simulink model "motorV1"  (R2022b)
settings: Solver=VariableStepAuto  StartTime=0.0  StopTime=10.0  RelTol=1e-3
undefined symbols (not defined in the file or in its folder): flux_a, flux_b, flux_c, Fx_idq, Fy_idq
settings Model: Creator=ramuj  LastModifiedBy=ramuj

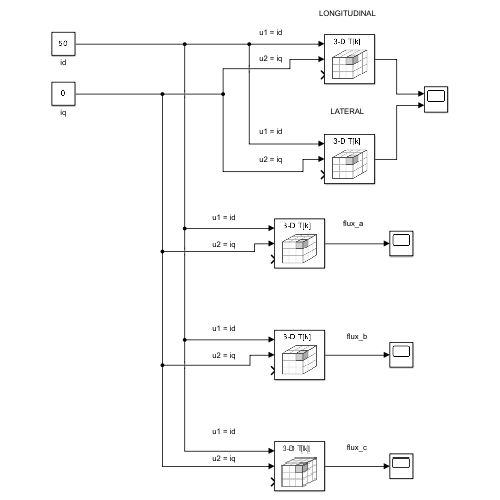
[thumbnail: Simulink's stored preview of the top-level diagram]
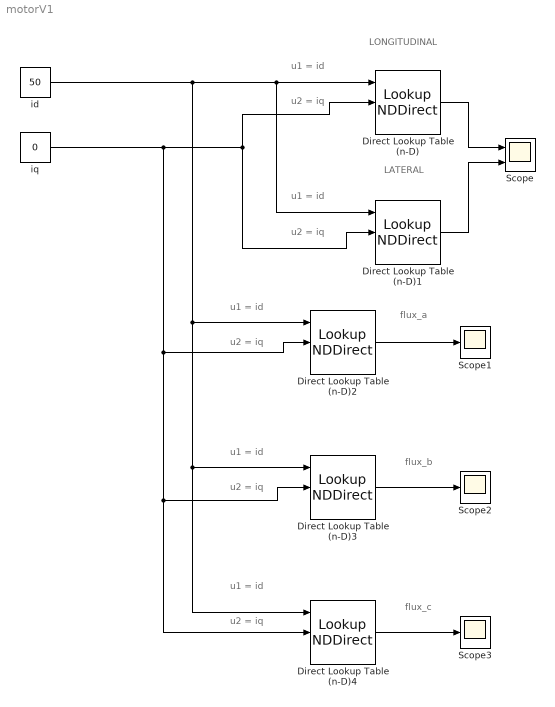
== system motorV1 ==
  note: flux_a
  note: u2 = iq
  note: u1 = id
  note: LONGITUDINAL
  note: LATERAL
  note: u1 = id
  note: u2 = iq
  note: u1 = id
  note: u2 = iq
  note: u2 = iq
  note: flux_b
  note: u1 = id
  note: flux_c
  note: u2 = iq
  note: u1 = id
  Direct Lookup Table (n-D) : LookupNDDirect  NumberOfTableDimensions=3  Table=Fx_idq
  Direct Lookup Table (n-D)1 : LookupNDDirect  NumberOfTableDimensions=3  Table=Fy_idq
  Direct Lookup Table (n-D)2 : LookupNDDirect  NumberOfTableDimensions=3  Table=flux_a
  Direct Lookup Table (n-D)3 : LookupNDDirect  NumberOfTableDimensions=3  Table=flux_b
  Direct Lookup Table (n-D)4 : LookupNDDirect  NumberOfTableDimensions=3  Table=flux_c
  Scope : Scope  NumInputPorts=2
  Scope1 : Scope
  Scope2 : Scope
  Scope3 : Scope
  id : Constant  Value=50
  iq : Constant  Value=0
  wires:
  Direct Lookup Table (n-D)/1 -> Scope/1
  Direct Lookup Table (n-D)1/1 -> Scope/2
  Direct Lookup Table (n-D)2/1 -> Scope1/1
  Direct Lookup Table (n-D)3/1 -> Scope2/1
  Direct Lookup Table (n-D)4/1 -> Scope3/1
  id/1 -> Direct Lookup Table (n-D)4/1, Direct Lookup Table (n-D)3/1, Direct Lookup Table (n-D)2/1, Direct Lookup Table (n-D)1/1, Direct Lookup Table (n-D)/1
  iq/1 -> Direct Lookup Table (n-D)1/2, Direct Lookup Table (n-D)/2, Direct Lookup Table (n-D)4/2, Direct Lookup Table (n-D)3/2, Direct Lookup Table (n-D)2/2
